simulink model "ACDCMG_woPV"  (R2020b)
settings: Solver=FixedStepAuto  StartTime=0.0  StopTime=0.2  FixedStep=Ts  MaxStep=1e-2  RelTol=1e-3
InitFcn:
  | Set_parameters_R2018
undefined symbols (not defined in the file): D1, D_invs, Delta, dis11, dis14, dis2, dis3, dis4, dis5, dis6, dis8, DiscIntNeverNeededParam, ee_sli_rtmsupport, fn, Fnom, gcbh, H_invs, Ion, Lithium, max_min, P_Load_3, P_nom_inv, Pnom_T1, Pnom_T2, Pnom_T3, Ql_Load_3, R_Load_9, R_Load_DC, Rl, Rls, S, sigbuilder_block, Ts, Ts_Control, Ts_Power, V1_LL_T3, VnInv, Vnom_DC, Vnom_Diesel, Vnom_prim, Vnom_sec, Vnom_ter_AC_DC, Xl, Xls
libraries: powerlib x238, powerlib_meascontrol x103, powerlib_extras x55, simulink x21, pid_lib x4, eeGeneralControl x2, re_lib x1, electricdrivelib x1, eeSinusoidalMeasurementV2 x1, eePowerMeasurement x1
(part 4 of 9)

== system ACDCMG_woPV/Resource1 ==
  note: http://calculationsolar.com/blog/?cat=2
  Constant1 : Constant  Value=max_min
  Irradiance (W/m^2) : Display
      settings: Format=bank  Decimation=1000
  Irradiance Temp Demand Max : Subsystem  Tag=STV Subsys  LoadFcn=sigbuilder_block('load');  StartFcn=sigbuilder_block('start');  StopFcn=sigbuilder_block('stop');  ClipboardFcn=sigbuilder_block('clipboard');  mask(Sigbuilder block){tuvar=[0:10]}
      mask help: Sigbuilder GUI
      mask init:
      | if ~strcmp(get_param(bdroot(gcbh),'SimulationStatus'),'stopped') tuvar = sigbuilder_block('maskInit'); end
      settings: CopyFcn=sigbuilder_block('copy');  DeleteFcn=sigbuilder_block('delete');  ModelCloseFcn=sigbuilder_block('modelClose');  PreSaveFcn=sigbuilder_block('preSave');  PauseFcn=sigbuilder_block('pause')  ContinueFcn=sigbuilder_block('continue')  NameChangeFcn=sigbuilder_block('namechange');  OpenFcn=sigbuilder_block('open',[0 30 1024.5 488.25 ]);  CloseFcn=sigbuilder_block('close');
      mask Display: plot(0, 0, 100, 100,[2, 2, 32, 32, 2], [68, 8, 8, 68, 68],[32, 2], [38, 38], [32, 19, 2],[53, 60, 44], [32, 17, 17, 2],[16, 16, 31, 31]);txt = getActiveGroup(gcbh);text(2, 100, txt,'verticalAlignment', 'top');
  Irradiance MIn Demand : Constant  Value=0
  Switch2 : Switch  Criteria=u2 > Threshold
  Temperature (deg. C) : Display
      settings: Format=bank  Decimation=1000
  Temp : Outport  VectorParamsAs1DForOutWhenUnconnected=off
  Ir : Outport  Port=2  VectorParamsAs1DForOutWhenUnconnected=off
  wires:
  Irradiance Temp Demand Max/1(Ir) -> Switch2/1, Irradiance (W/m^2)/1
  Irradiance Temp Demand Max/2(Temp) -> Temp/1, Temperature (deg. C)/1
  Irradiance MIn Demand/1 -> Switch2/3
  Constant1/1 -> Switch2/2
  Switch2/1 -> Ir/1  "Radiación (kW/m2)"

== system ACDCMG_woPV/Boost -buck Bi-directional converter 1 0.65 kW/+ve reference For Buck --> -ve reference For Boost <-- ==
  note: Buck PWM
  note: Duty Cycle
  note: Upper logic
  note: Lower logic
  note: Boost PWM
  note: Duty Cycle
  I_ref : Inport
  PID Orig Boost : Subsystem
  PID Orig Buck : Subsystem
  Relational Operator : RelationalOperator  Operator=>  OutDataTypeStr=boolean  RndMeth=Nearest
  Relational Operator1 : RelationalOperator  Operator=>  OutDataTypeStr=boolean  RndMeth=Nearest
  Saturation : Saturate  UpperLimit=0.9  LowerLimit=0
  Saturation1 : Saturate  UpperLimit=0.8  LowerLimit=0
  Sawtooth : simulink/Sources/Repeating Sequence  rep_seq_t=[0 1/5000]  rep_seq_y=[0 1]
  Sawtooth1 : simulink/Sources/Repeating Sequence  rep_seq_t=[0 1/5000]  rep_seq_y=[0 1]
  Sign : Gain  Gain=-1
  Sign1 : Gain  Gain=-1
  Sum : Sum  Inputs=|+-
  Sum2 : Sum  Inputs=-+|
  Switch : Switch  Criteria=u2 > Threshold
  Switch1 : Switch
  Vref1 : Constant  Value=0
  Vref2 : Constant  Value=0
  buck_I_Ctrl : Outport  VectorParamsAs1DForOutWhenUnconnected=off
  boost_I_Ctrl : Outport  Port=2  VectorParamsAs1DForOutWhenUnconnected=off
  wires:
  Sum/1 -> PID Orig Boost/1(error)  "error"
  Relational Operator/1 -> [boost1]
  Sign/1 -> Sum/1
  PID Orig Boost/1(Out1) -> Saturation/1
  PID Orig Buck/1(Out1) -> Saturation1/1
  Sawtooth/1 -> Relational Operator/2
  Sawtooth1/1 -> Relational Operator1/2
  Relational Operator1/1 -> [buck1]
  Sum2/1 -> PID Orig Buck/1(error)  "error"
  Saturation/1 -> Relational Operator/1
  Saturation1/1 -> Relational Operator1/1
  Vref1/1 -> Switch/3
  Vref2/1 -> Switch1/1
  [boost1] -> Switch1/3
  [buck1] -> Switch/1
  I_ref/1 -> Switch1/2, Switch/2, Sum2/2, Sign/1  "Current Reference"
  Sign1/1 -> Sum/2
  Switch1/1 -> boost_I_Ctrl/1
  Switch/1 -> buck_I_Ctrl/1
  [current] -> Sum2/1, Sign1/1

== system ACDCMG_woPV/Boost -buck Bi-directional converter 1 0.65 kW/OP_max // min ==
  boost_V_Ctrll : Inport
  buck_V_Ctrl : Inport  Port=2
  buck_I_Ctrl : Inport  Port=3
  boost_I_Ctrll : Inport  Port=4
  Control modes 0- Current 1- Coltage : Constant
  OP_max1 : Constant
  OP_min1 : Constant  Value=0
  Switch1 : Switch  Criteria=u2 > Threshold
  Switch2 : Switch  Criteria=u2 > Threshold
  Switch3 : Switch  Criteria=u2 > Threshold
  Op_Max / Min : Outport  VectorParamsAs1DForOutWhenUnconnected=off
  g_buck : Outport  Port=2  VectorParamsAs1DForOutWhenUnconnected=off
  g_boost : Outport  Port=3  VectorParamsAs1DForOutWhenUnconnected=off
  wires:
  OP_max1/1 -> Switch2/1
  OP_min1/1 -> Switch2/3
  Switch2/1 -> Op_Max / Min/1
  Control modes 0- Current 1- Coltage/1 -> Switch2/2, Switch1/2, Switch3/2
  boost_I_Ctrll/1 -> Switch1/3
  boost_V_Ctrll/1 -> Switch1/1
  buck_V_Ctrl/1 -> Switch3/1
  buck_I_Ctrl/1 -> Switch3/3
  Switch1/1 -> g_boost/1
  Switch3/1 -> g_buck/1

== system ACDCMG_woPV/Boost -buck Bi-directional converter 1 0.65 kW/Primary Control ==
  V_ref : Inport
  Constant : Constant
  Display3 : Display  Commented=on
  From1 : From  Commented=on  GotoTag=Vdc_bus  TagVisibility=global
  From4 : From  Commented=on  GotoTag=boost1
  From5 : From  Commented=on  GotoTag=buck1
  PID Orig Boost : Subsystem
  Relational Operator2 : RelationalOperator  Commented=on  Operator=>  OutDataTypeStr=boolean  RndMeth=Nearest
  Saturation : Saturate  UpperLimit=0.9  LowerLimit=0.1
  Scope1 : Scope
  Sum : Sum  Inputs=|+-
  Sum1 : Sum  Inputs=|-+
  Switch : Switch  Commented=on  Criteria=u2 > Threshold  Threshold=300
  Switch1 : Switch  Commented=on  Criteria=u2 > Threshold  Threshold=300
  Vref1 : Constant  Commented=on  Value=0
  Vref2 : Constant  Commented=on  Value=0
  Duty_Ctrl : Outport  VectorParamsAs1DForOutWhenUnconnected=off
  Comp_Duty_Ctrl : Outport  Port=2  VectorParamsAs1DForOutWhenUnconnected=off
  wires:
  Relational Operator2/1 -> Switch1/2, Switch/2
  V_ref/1 -> Sum/1, Relational Operator2/2
  From1/1 -> Relational Operator2/1
  Vref2/1 -> Switch1/1
  [Vdc_bus] -> Sum/2
  From5/1 -> Switch/1
  From4/1 -> Switch1/3
  Switch/1 -> Display3/1
  Vref1/1 -> Switch/3
  Sum/1 -> PID Orig Boost/1(error)  "error"
  PID Orig Boost/1(Out1) -> Saturation/1
  Constant/1 -> Sum1/2
  Saturation/1 -> Sum1/1, Duty_Ctrl/1, Scope1/1
  Sum1/1 -> Comp_Duty_Ctrl/1

== system ACDCMG_woPV/Boost -buck Bi-directional converter DC //CD 1 0.65 kW/+ve reference For Buck --> -ve reference For Boost <-- ==
  note: Notes :
      | 1- Saturation block : in practical applications during experiment, in the begining if the experiment, the error is usually high, therefore, duty cycle might reach value of 1, which means the IGBT switch will be shorted for a while which might cause damage to your circuit. it is preferable to put the saturation value to 0.7 during experiment, once you trust your circuit, you can increase up to 0.9.
      | 2- Sawtooth : We choose the frequancy of the sawtooth to be 5 kHz, because according to some papers if you go beyond this value, parastic elements will show up (i.e. its like an imaginary resistance and capcitance that causes switching losses and heat). But the more you increase the frequency, the smoother the signal you will get.
      | 3- Step size of your mode l: Make sure that the step size (sample time) in the "model configuration parameters" is smaller than 1/f of the sawtooth. For example, lets say that the sawtooth f = 2 Hz or cycle/sec, meaning the triangle (cycle) repeats every 1/2 sec. Step size or sample time means how many point matlab plot every cycle, lets say it is 1/4 (i.e. plot a point every 0.25 sec), that means that the triangle will be plotted with only two points. That reduce the accuracy, Moreover if the step size is greater than 1/f of the sawtooth, the sawtooth output will be zero.
  note: Buck PWM
  note: Duty Cycle
  note: Upper logic
  note: Lower logic
  note: Boost PWM
  note: Duty Cycle
  I_ref : Inport
  Display3 : Display
  Display4 : Display
  Integrator : Integrator  LimitOutput=on  UpperSaturationLimit=0.9  LowerSaturationLimit=0
  Integrator1 : Integrator  LimitOutput=on  UpperSaturationLimit=0.9  LowerSaturationLimit=0
  Ki : Gain  Gain=3
  Ki1 : Gain  Gain=110
  Kp : Gain  Gain=0.02
  Kp1 : Gain  Gain=0.2
  Relational Operator : RelationalOperator  Operator=>  OutDataTypeStr=boolean  RndMeth=Nearest
  Relational Operator1 : RelationalOperator  Operator=>  OutDataTypeStr=boolean  RndMeth=Nearest
  Saturation : Saturate  UpperLimit=0.9  LowerLimit=0
  Saturation1 : Saturate  UpperLimit=0.8  LowerLimit=0
  Sawtooth : simulink/Sources/Repeating Sequence  rep_seq_t=[0 1/5000]  rep_seq_y=[0 1]
  Sawtooth1 : simulink/Sources/Repeating Sequence  rep_seq_t=[0 1/5000]  rep_seq_y=[0 1]
  Sign : Gain  Gain=-1
  Sign1 : Gain  Gain=-1
  Sum : Sum  Inputs=|+-
  Sum1 : Sum  Inputs=|++
  Sum2 : Sum  Inputs=|+-
  Sum3 : Sum  Inputs=|++
  Switch : Switch  Criteria=u2 > Threshold
  Switch1 : Switch
  Vref1 : Constant  Value=0
  Vref2 : Constant  Value=0
  buck : Outport  VectorParamsAs1DForOutWhenUnconnected=off
  boost : Outport  Port=2  VectorParamsAs1DForOutWhenUnconnected=off
  tag scope: boost1=global, buck1=global
  wires:
  Integrator/1 -> Sum1/2
  Kp/1 -> Sum1/1
  Sum/1 -> Kp/1, Ki/1  "error"
  Relational Operator/1 -> [boost1]
  Sign/1 -> Sum/1
  Sum1/1 -> Saturation/1
  Ki/1 -> Integrator/1
  Sum3/1 -> Saturation1/1
  Integrator1/1 -> Sum3/2
  Sawtooth/1 -> Relational Operator/2
  Sawtooth1/1 -> Relational Operator1/2
  [current] -> Sum2/2, Sign1/1
  Kp1/1 -> Sum3/1
  Relational Operator1/1 -> [buck1]
  Sum2/1 -> Ki1/1, Kp1/1  "error"
  Saturation/1 -> Relational Operator/1
  Saturation1/1 -> Relational Operator1/1
  Ki1/1 -> Integrator1/1
  Vref1/1 -> Switch/3
  Vref2/1 -> Switch1/1
  [boost1] -> Switch1/3
  [buck1] -> Switch/1
  I_ref/1 -> Sum2/1, Sign/1, Switch1/2, Switch/2  "Current Reference"
  Sign1/1 -> Sum/2
  Switch1/1 -> Display4/1, boost/1
  Switch/1 -> Display3/1, buck/1

== system ACDCMG_woPV/Boost -buck Bi-directional converter DC //CD 1 0.65 kW/ref ==
  note: 1 -charge
      | 0-discharge
  Constant2 : Constant  Value=max_min
  Constant3 : Constant  Value=max_min
  Current reference (battery charge) OP_Max : Constant  Value=5
  Current reference (battery discharge) OP_Max1 : Constant  Value=-5
  Min Demand OP_min : Constant  Value=3
  Min Demand OP_min1 : Constant  Value=-3
  Switch : Switch  Criteria=u2 > Threshold
  Switch1 : Switch  Criteria=u2 > Threshold
  Switch3 : Switch  Criteria=u2 > Threshold
  Vref1 : Constant
  ref : Outport  VectorParamsAs1DForOutWhenUnconnected=off
  wires:
  Constant3/1 -> Switch3/2
  Switch3/1 -> Switch/3
  Switch1/1 -> Switch/1
  Vref1/1 -> Switch/2
  Min Demand OP_min/1 -> Switch1/3
  Current reference (battery charge) OP_Max/1 -> Switch1/1
  Min Demand OP_min1/1 -> Switch3/3
  Constant2/1 -> Switch1/2
  Current reference (battery discharge) OP_Max1/1 -> Switch3/1
  Switch/1 -> ref/1

== system ACDCMG_woPV/Boost -buck Bi-directional converter DC //DC 1 0.65 kW Switching Model/+ve reference For Buck --> -ve reference For Boost <-- ==
  note: Buck PWM
  note: Duty Cycle
  note: Upper logic
  note: Lower logic
  note: Boost PWM
  note: Duty Cycle
  I_ref : Inport
  PID Orig Boost : Subsystem
  PID Orig Buck : Subsystem
  Relational Operator : RelationalOperator  Operator=>  OutDataTypeStr=boolean  RndMeth=Nearest
  Relational Operator1 : RelationalOperator  Operator=>  OutDataTypeStr=boolean  RndMeth=Nearest
  Saturation : Saturate  UpperLimit=0.9  LowerLimit=0
  Saturation1 : Saturate  UpperLimit=0.8  LowerLimit=0
  Sawtooth : simulink/Sources/Repeating Sequence  rep_seq_t=[0 1/5000]  rep_seq_y=[0 1]
  Sawtooth1 : simulink/Sources/Repeating Sequence  rep_seq_t=[0 1/5000]  rep_seq_y=[0 1]
  Sign : Gain  Gain=-1
  Sign1 : Gain  Gain=-1
  Sum : Sum  Inputs=|+-
  Sum2 : Sum  Inputs=-+|
  Switch : Switch  Criteria=u2 > Threshold
  Switch1 : Switch
  Vref1 : Constant  Value=0
  Vref2 : Constant  Value=0
  buck_I_Ctrl : Outport  VectorParamsAs1DForOutWhenUnconnected=off
  boost_I_Ctrl : Outport  Port=2  VectorParamsAs1DForOutWhenUnconnected=off
  wires:
  Sum/1 -> PID Orig Boost/1(error)  "error"
  Relational Operator/1 -> [boost1]
  Sign/1 -> Sum/1
  PID Orig Boost/1(Out1) -> Saturation/1
  PID Orig Buck/1(Out1) -> Saturation1/1
  Sawtooth/1 -> Relational Operator/2
  Sawtooth1/1 -> Relational Operator1/2
  Relational Operator1/1 -> [buck1]
  Sum2/1 -> PID Orig Buck/1(error)  "error"
  Saturation/1 -> Relational Operator/1
  Saturation1/1 -> Relational Operator1/1
  Vref1/1 -> Switch/3
  Vref2/1 -> Switch1/1
  [boost1] -> Switch1/3
  [buck1] -> Switch/1
  I_ref/1 -> Switch1/2, Switch/2, Sum2/2, Sign/1  "Current Reference"
  Sign1/1 -> Sum/2
  Switch1/1 -> boost_I_Ctrl/1
  Switch/1 -> buck_I_Ctrl/1
  [current] -> Sum2/1, Sign1/1

== system ACDCMG_woPV/Boost -buck Bi-directional converter DC //DC 1 0.65 kW Switching Model/OP_max // min ==
  boost_V_Ctrll : Inport
  buck_V_Ctrl : Inport  Port=2
  buck_I_Ctrl : Inport  Port=3
  boost_I_Ctrll : Inport  Port=4
  Control modes 0- Current 1- Coltage : Constant
  OP_max1 : Constant
  OP_min1 : Constant  Value=0
  Switch1 : Switch  Criteria=u2 > Threshold
  Switch2 : Switch  Criteria=u2 > Threshold
  Switch3 : Switch  Criteria=u2 > Threshold
  Op_Max / Min : Outport  VectorParamsAs1DForOutWhenUnconnected=off
  g_buck : Outport  Port=2  VectorParamsAs1DForOutWhenUnconnected=off
  g_boost : Outport  Port=3  VectorParamsAs1DForOutWhenUnconnected=off
  wires:
  OP_max1/1 -> Switch2/1
  OP_min1/1 -> Switch2/3
  Switch2/1 -> Op_Max / Min/1
  Control modes 0- Current 1- Coltage/1 -> Switch2/2, Switch1/2, Switch3/2
  boost_I_Ctrll/1 -> Switch1/3
  boost_V_Ctrll/1 -> Switch1/1
  buck_V_Ctrl/1 -> Switch3/1
  buck_I_Ctrl/1 -> Switch3/3
  Switch1/1 -> g_boost/1
  Switch3/1 -> g_buck/1

== system ACDCMG_woPV/Boost -buck Bi-directional converter DC //DC 1 0.65 kW Switching Model/Primary Control ==
  V_ref : Inport
  Display3 : Display
  Display4 : Display
  PID Orig Boost : Subsystem
  PID Orig Buck : Subsystem
  Relational Operator : RelationalOperator  Operator=>  OutDataTypeStr=boolean  RndMeth=Nearest
  Relational Operator1 : RelationalOperator  Operator=>  OutDataTypeStr=boolean  RndMeth=Nearest
  Relational Operator2 : RelationalOperator  Operator=>  OutDataTypeStr=boolean  RndMeth=Nearest
  Repeating Sequence : simulink/Sources/Repeating Sequence  rep_seq_t=[0 1/5000]  rep_seq_y=[0 1]
  Repeating Sequence1 : simulink/Sources/Repeating Sequence  rep_seq_t=[0 1/5000]  rep_seq_y=[0 1]
  Saturation : Saturate  UpperLimit=0.9  LowerLimit=0
  Saturation1 : Saturate  UpperLimit=0.9  LowerLimit=0
  Sum : Sum  Inputs=|+-
  Sum2 : Sum  Inputs=|+-
  Switch : Switch  Criteria=u2 > Threshold  Threshold=300
  Switch1 : Switch  Criteria=u2 > Threshold  Threshold=300
  Vref1 : Constant  Value=0
  Vref2 : Constant  Value=0
  buck_V_Ctrl : Outport  VectorParamsAs1DForOutWhenUnconnected=off
  boost_V_Ctrl : Outport  Port=2  VectorParamsAs1DForOutWhenUnconnected=off
  wires:
  Relational Operator2/1 -> Switch1/2, Switch/2
  Saturation1/1 -> Relational Operator1/1
  V_ref/1 -> Sum/1, Relational Operator2/2, Sum2/1
  [Vdc_bus] -> Relational Operator2/1
  Vref2/1 -> Switch1/1
  Repeating Sequence/1 -> Relational Operator/2
  Repeating Sequence1/1 -> Relational Operator1/2
  Relational Operator1/1 -> [buck1]
  [Vdc_bus] -> Sum2/2, Sum/2
  [buck1] -> Switch/1
  Switch1/1 -> Display4/1, boost_V_Ctrl/1
  Saturation/1 -> Relational Operator/1
  [boost1] -> Switch1/3
  Sum2/1 -> PID Orig Buck/1(error)  "error"
  Relational Operator/1 -> [boost1]
  Switch/1 -> Display3/1, buck_V_Ctrl/1
  Vref1/1 -> Switch/3
  Sum/1 -> PID Orig Boost/1(error)  "error"
  PID Orig Buck/1(Out1) -> Saturation1/1
  PID Orig Boost/1(Out1) -> Saturation/1

== system ACDCMG_woPV/Boost converter DC //CD 2 5 kHz - 300V /MPPT Controller using  "Incremental Conductance + Integral Regulator "  technique  ==
  note: +
  note: control mppt
  V_PV : Inport
  I_PV : Inport  Port=2
  Add : Sum  Inputs=+-
  Deblock MPPT : Step  Time=0.2  SampleTime=0
  Duty Cycle : Constant  Value=Dinit
  MPPT : Subsystem
  PWM Generator (DC-DC) : powerlib_meascontrol/Pulse & Signal Generators/PWM Generator (DC-DC)  Fsw=fc  Ts=Ts_Power
  Saturation : Saturate  UpperLimit=1  LowerLimit=0
  Pulses : Outport  VectorParamsAs1DForOutWhenUnconnected=off
  tag scope: D=global
  wires:
  V_PV/1 -> MPPT/1(V_PV)
  I_PV/1 -> MPPT/2(I_PV)
  PWM Generator (DC-DC)/1 -> Pulses/1
  Deblock MPPT/1 -> MPPT/3(on/off)
  Add/1 -> Saturation/1  "D"
  MPPT/1(Delta_D) -> Add/2  "Vdc_ref"
  Duty Cycle/1 -> Add/1
  Saturation/1 -> [D], PWM Generator (DC-DC)/1

== system ACDCMG_woPV/Boost converter DC //CD 2 5 kHz - 300V 1/MPPT Controller using  "Incremental Conductance + Integral Regulator "  technique  ==
  note: +
  note: control mppt
  V_PV : Inport
  I_PV : Inport  Port=2
  Add : Sum  Inputs=+-
  Deblock MPPT : Step  Time=0.2  SampleTime=0
  Duty Cycle : Constant  Value=Dinit
  MPPT : Subsystem
  PWM Generator (DC-DC) : powerlib_meascontrol/Pulse & Signal Generators/PWM Generator (DC-DC)  Fsw=fc  Ts=Ts_Power
  Saturation : Saturate  UpperLimit=1  LowerLimit=0
  Pulses : Outport  VectorParamsAs1DForOutWhenUnconnected=off
  tag scope: D=global
  wires:
  V_PV/1 -> MPPT/1(V_PV)
  I_PV/1 -> MPPT/2(I_PV)
  PWM Generator (DC-DC)/1 -> Pulses/1
  Deblock MPPT/1 -> MPPT/3(on/off)
  Add/1 -> Saturation/1  "D"
  MPPT/1(Delta_D) -> Add/2  "Vdc_ref"
  Duty Cycle/1 -> Add/1
  Saturation/1 -> [D], PWM Generator (DC-DC)/1

== system ACDCMG_woPV/Boost converter DC //DC 2 5 kHz - 300V /  ==
  V_PV : Inport
  I_PV : Inport  Port=2
  Duty Cycle : Constant  Value=0.34
  PWM Generator (DC-DC) : powerlib_meascontrol/Pulse & Signal Generators/PWM Generator (DC-DC)  Fsw=fc  Ts=Ts_Power
  Terminator1 : Terminator
  Terminator2 : Terminator
  Pulses : Outport  VectorParamsAs1DForOutWhenUnconnected=off
  tag scope: D=global
  wires:
  V_PV/1 -> Terminator1/1
  I_PV/1 -> Terminator2/1
  PWM Generator (DC-DC)/1 -> Pulses/1
  Duty Cycle/1 -> [D], PWM Generator (DC-DC)/1

== system ACDCMG_woPV/Bus_1/Power Factor Block1 ==
  Vabc : Inport
  Iabc : Inport  Port=2
  Complex to Magnitude-Angle : ComplexToMagnitudeAngle  Commented=on
  Conv pu1 : Gain  Gain=sqrt (3) /Vnom_sec  SaturateOnIntegerOverflow=on  OutDataTypeStr=Inherit: Same as input  ParamDataTypeStr=Inherit: Same as input
  Current1 : Goto  Commented=on  GotoTag=P_abc_Bus1  TagVisibility=global
  Current2 : Goto  Commented=on  GotoTag=Q_abc_Bus1  TagVisibility=global
  Gain1 : Gain  Commented=on  Gain=-1/1000
  Mux : Mux  Inputs=2
  Power : powerlib_meascontrol/Measurements/Power  Commented=on  Freq=Freq  Vinit=Vinit  Iinit=Iinit  Ts=Ts
  Real-Imag to Complex : RealImagToComplex  Commented=on
  Terminator : Terminator  Commented=on
  cos(theta) : Trigonometry  Commented=on  Operator=cos
  to Kw : Gain  Commented=on  Gain=-1/1000
  "Vabc y Vabc " : Outport  VectorParamsAs1DForOutWhenUnconnected=off
  "Iabc y Iabc " : Outport  Port=2  VectorParamsAs1DForOutWhenUnconnected=off
  tag scope: Vabc_LL_pu_Bus1=global
  wires:
  Power/1 -> Gain1/1, Real-Imag to Complex/1
  Power/2 -> Real-Imag to Complex/2, to Kw/1
  Complex to Magnitude-Angle/2 -> cos(theta)/1
  Real-Imag to Complex/1 -> Complex to Magnitude-Angle/1
  Complex to Magnitude-Angle/1 -> Terminator/1
  Iabc/1 -> "Iabc y Iabc "/1, Power/2
  Mux/1 -> "Vabc y Vabc "/1
  Vabc/1 -> Power/1, Conv pu1/1, Mux/1, Mux/2
  Conv pu1/1 -> [Vabc_LL_pu_Bus1]
  to Kw/1 -> Current2/1
  Gain1/1 -> Current1/1

== system ACDCMG_woPV/Bus_2/Power Factor Block1 ==
  Vabc : Inport
  Iabc : Inport  Port=2
  Complex to Magnitude-Angle : ComplexToMagnitudeAngle  Commented=on
  Conv pu1 : Gain  Gain=sqrt (3) /Vnom_sec  SaturateOnIntegerOverflow=on  OutDataTypeStr=Inherit: Same as input  ParamDataTypeStr=Inherit: Same as input
  Current3 : Goto  Commented=on  GotoTag=P_abc_Bus2  TagVisibility=global
  Current4 : Goto  Commented=on  GotoTag=Q_abc_Bus2  TagVisibility=global
  Mux : Mux  Inputs=2
  Power : powerlib_meascontrol/Measurements/Power  Commented=on  Freq=Freq  Vinit=Vinit  Iinit=Iinit  Ts=Ts
  Real-Imag to Complex : RealImagToComplex  Commented=on
  Terminator : Terminator  Commented=on
  cos(theta) : Trigonometry  Commented=on  Operator=cos
  to Kw : Gain  Commented=on  Gain=-1/1000
  to Kw1 : Gain  Commented=on  Gain=-1/1000
  "Vabc y Vabc " : Outport  VectorParamsAs1DForOutWhenUnconnected=off
  Iabc y Iabc : Outport  Port=2  VectorParamsAs1DForOutWhenUnconnected=off
  tag scope: Vabc_LL_pu_Bus2=global
  wires:
  Complex to Magnitude-Angle/2 -> cos(theta)/1
  Real-Imag to Complex/1 -> Complex to Magnitude-Angle/1
  cos(theta)/1 -> ?
  Complex to Magnitude-Angle/1 -> Terminator/1
  Iabc/1 -> Iabc y Iabc/1, Power/2
  Mux/1 -> "Vabc y Vabc "/1
  Vabc/1 -> Power/1, Conv pu1/1, Mux/1, Mux/2
  Conv pu1/1 -> [Vabc_LL_pu_Bus2]
  Power/1 -> to Kw1/1, Real-Imag to Complex/1
  Power/2 -> to Kw/1, Real-Imag to Complex/2
  to Kw/1 -> Current4/1
  to Kw1/1 -> Current3/1

== system ACDCMG_woPV/Bus_3 /Power Factor Block1 ==
  Vabc : Inport
  Iabc : Inport  Port=2
  Complex to Magnitude-Angle : ComplexToMagnitudeAngle  Commented=on
  Conv pu2 : Gain  Gain=sqrt (3) /Vnom_prim  SaturateOnIntegerOverflow=on  OutDataTypeStr=Inherit: Same as input  ParamDataTypeStr=Inherit: Same as input
  Current3 : Goto  Commented=on  GotoTag=P_abc_Bus3  TagVisibility=global
  Current4 : Goto  Commented=on  GotoTag=Q_abc_Bus3  TagVisibility=global
  Gain : Gain  Commented=on  Gain=-1/1000
  Gain1 : Gain  Commented=on  Gain=-1/1000
  Mux : Mux  Inputs=2
  Power : powerlib_meascontrol/Measurements/Power  Commented=on  Freq=Freq  Vinit=Vinit  Iinit=Iinit  Ts=Ts
  Real-Imag to Complex : RealImagToComplex  Commented=on
  Terminator : Terminator  Commented=on
  cos(theta) : Trigonometry  Commented=on  Operator=cos
  "Vabc y Vabc " : Outport  VectorParamsAs1DForOutWhenUnconnected=off
  "Iabc y Iabc " : Outport  Port=2  VectorParamsAs1DForOutWhenUnconnected=off
  tag scope: Vabc_LL_pu_Bus3=global
  wires:
  Complex to Magnitude-Angle/2 -> cos(theta)/1
  Real-Imag to Complex/1 -> Complex to Magnitude-Angle/1
  cos(theta)/1 -> ?
  Complex to Magnitude-Angle/1 -> Terminator/1
  Iabc/1 -> "Iabc y Iabc "/1, Power/2
  Mux/1 -> "Vabc y Vabc "/1
  Vabc/1 -> Power/1, Conv pu2/1, Mux/1, Mux/2
  Conv pu2/1 -> [Vabc_LL_pu_Bus3]
  Power/1 -> Gain/1, Real-Imag to Complex/1
  Power/2 -> Real-Imag to Complex/2, Gain1/1
  Gain1/1 -> Current4/1
  Gain/1 -> Current3/1

== system ACDCMG_woPV/Bus_4/Power Factor Block1 ==
  Vabc : Inport
  Iabc : Inport  Port=2
  Complex to Magnitude-Angle : ComplexToMagnitudeAngle  Commented=on
  Conv pu1 : Gain  Gain=sqrt (3) /Vnom_sec  SaturateOnIntegerOverflow=on  OutDataTypeStr=Inherit: Same as input  ParamDataTypeStr=Inherit: Same as input
  Current3 : Goto  Commented=on  GotoTag=P_abc_Bus4  TagVisibility=global
  Current4 : Goto  Commented=on  GotoTag=Q_abc_Bus4  TagVisibility=global
  Mux : Mux  Inputs=2
  Power : powerlib_meascontrol/Measurements/Power  Commented=on  Freq=Freq  Vinit=Vinit  Iinit=Iinit  Ts=Ts
  Real-Imag to Complex : RealImagToComplex  Commented=on
  Terminator : Terminator  Commented=on
  cos(theta) : Trigonometry  Commented=on  Operator=cos
  to Kw : Gain  Commented=on  Gain=1/1000
  to Kw1 : Gain  Commented=on  Gain=1/1000
  Vabc y Vabc : Outport  VectorParamsAs1DForOutWhenUnconnected=off
  "Iabc y Iabc " : Outport  Port=2  VectorParamsAs1DForOutWhenUnconnected=off
  tag scope: Vabc_LL_pu_Bus4=global
  wires:
  Complex to Magnitude-Angle/2 -> cos(theta)/1
  Real-Imag to Complex/1 -> Complex to Magnitude-Angle/1
  cos(theta)/1 -> ?
  Complex to Magnitude-Angle/1 -> Terminator/1
  Iabc/1 -> "Iabc y Iabc "/1, Power/2
  Mux/1 -> Vabc y Vabc/1
  Conv pu1/1 -> [Vabc_LL_pu_Bus4]
  Vabc/1 -> Power/1, Conv pu1/1, Mux/1, Mux/2
  Power/2 -> Real-Imag to Complex/2, to Kw/1
  Power/1 -> to Kw1/1, Real-Imag to Complex/1
  to Kw/1 -> Current4/1
  to Kw1/1 -> Current3/1

== system ACDCMG_woPV/Bus_5/Power Factor Block1 ==
  Vabc : Inport
  Iabc : Inport  Port=2
  Complex to Magnitude-Angle : ComplexToMagnitudeAngle  Commented=on
  Conv pu1 : Gain  Gain=sqrt (3) /Vnom_sec  SaturateOnIntegerOverflow=on  OutDataTypeStr=Inherit: Same as input  ParamDataTypeStr=Inherit: Same as input
  Current3 : Goto  Commented=on  GotoTag=P_abc_Bus5  TagVisibility=global
  Current4 : Goto  Commented=on  GotoTag=Q_abc_Bus5  TagVisibility=global
  Mux : Mux  Inputs=2
  Power : powerlib_meascontrol/Measurements/Power  Commented=on  Freq=Freq  Vinit=Vinit  Iinit=Iinit  Ts=Ts
  Real-Imag to Complex : RealImagToComplex  Commented=on
  Terminator : Terminator  Commented=on
  cos(theta) : Trigonometry  Commented=on  Operator=cos
  to Kw : Gain  Commented=on  Gain=1/1000
  to Kw1 : Gain  Commented=on  Gain=1/1000
  Vabc y Vabc : Outport  VectorParamsAs1DForOutWhenUnconnected=off
  "Iabc y Iabc " : Outport  Port=2  VectorParamsAs1DForOutWhenUnconnected=off
  tag scope: Vabc_LL_pu_Bus5=global
  wires:
  Complex to Magnitude-Angle/2 -> cos(theta)/1
  Real-Imag to Complex/1 -> Complex to Magnitude-Angle/1
  cos(theta)/1 -> ?
  Complex to Magnitude-Angle/1 -> Terminator/1
  Iabc/1 -> "Iabc y Iabc "/1, Power/2
  Mux/1 -> Vabc y Vabc/1
  Conv pu1/1 -> [Vabc_LL_pu_Bus5]
  Vabc/1 -> Power/1, Conv pu1/1, Mux/1, Mux/2
  Power/2 -> Real-Imag to Complex/2, to Kw/1
  Power/1 -> to Kw1/1, Real-Imag to Complex/1
  to Kw/1 -> Current4/1
  to Kw1/1 -> Current3/1

== system ACDCMG_woPV/Bus_6/Power Factor Block1 ==
  Vabc : Inport
  Iabc : Inport  Port=2
  Complex to Magnitude-Angle : ComplexToMagnitudeAngle  Commented=on
  Conv pu2 : Gain  Gain=sqrt (3) /Vnom_prim  SaturateOnIntegerOverflow=on  OutDataTypeStr=Inherit: Same as input  ParamDataTypeStr=Inherit: Same as input
  Current3 : Goto  Commented=on  GotoTag=P_abc_Bus6  TagVisibility=global
  Current4 : Goto  Commented=on  GotoTag=Q_abc_Bus6  TagVisibility=global
  Mux : Mux  Inputs=2
  Power : powerlib_meascontrol/Measurements/Power  Commented=on  Freq=Freq  Vinit=Vinit  Iinit=Iinit  Ts=Ts
  Real-Imag to Complex : RealImagToComplex  Commented=on
  Terminator : Terminator  Commented=on
  cos(theta) : Trigonometry  Commented=on  Operator=cos
  to Kw : Gain  Commented=on  Gain=1/1000
  to Kw1 : Gain  Commented=on  Gain=1/1000
  "Vabc y Vabc " : Outport  VectorParamsAs1DForOutWhenUnconnected=off
  "Iabc y Iabc " : Outport  Port=2  VectorParamsAs1DForOutWhenUnconnected=off
  tag scope: Vabc_LL_pu_Bus6=global
  wires:
  Complex to Magnitude-Angle/2 -> cos(theta)/1
  Real-Imag to Complex/1 -> Complex to Magnitude-Angle/1
  cos(theta)/1 -> ?
  Complex to Magnitude-Angle/1 -> Terminator/1
  Iabc/1 -> "Iabc y Iabc "/1, Power/2
  Mux/1 -> "Vabc y Vabc "/1
  Vabc/1 -> Power/1, Conv pu2/1, Mux/1, Mux/2
  Conv pu2/1 -> [Vabc_LL_pu_Bus6]
  Power/2 -> Real-Imag to Complex/2, to Kw/1
  Power/1 -> to Kw1/1, Real-Imag to Complex/1
  to Kw/1 -> Current4/1
  to Kw1/1 -> Current3/1

== system ACDCMG_woPV/Bus_7/Power Factor Block1 ==
  Vabc : Inport
  Iabc : Inport  Port=2
  Complex to Magnitude-Angle : ComplexToMagnitudeAngle  Commented=on
  Conv pu2 : Gain  Gain=sqrt (3) /Vnom_prim  SaturateOnIntegerOverflow=on  OutDataTypeStr=Inherit: Same as input  ParamDataTypeStr=Inherit: Same as input
  Current3 : Goto  Commented=on  GotoTag=P_abc_Bus7  TagVisibility=global
  Current4 : Goto  Commented=on  GotoTag=Q_abc_Bus7  TagVisibility=global
  Mux : Mux  Inputs=2
  Power : powerlib_meascontrol/Measurements/Power  Commented=on  Freq=Freq  Vinit=Vinit  Iinit=Iinit  Ts=Ts
  Real-Imag to Complex : RealImagToComplex  Commented=on
  Terminator : Terminator  Commented=on
  cos(theta) : Trigonometry  Commented=on  Operator=cos
  to Kw : Gain  Commented=on  Gain=1/1000
  to Kw1 : Gain  Commented=on  Gain=1/1000
  "Vabc y Vabc " : Outport  VectorParamsAs1DForOutWhenUnconnected=off
  "Iabc y Iabc " : Outport  Port=2  VectorParamsAs1DForOutWhenUnconnected=off
  tag scope: Vabc_LL_pu_Bus7=global
  wires:
  Complex to Magnitude-Angle/2 -> cos(theta)/1
  Real-Imag to Complex/1 -> Complex to Magnitude-Angle/1
  cos(theta)/1 -> ?
  Complex to Magnitude-Angle/1 -> Terminator/1
  Iabc/1 -> "Iabc y Iabc "/1, Power/2
  Mux/1 -> "Vabc y Vabc "/1
  Conv pu2/1 -> [Vabc_LL_pu_Bus7]
  Vabc/1 -> Power/1, Conv pu2/1, Mux/1, Mux/2
  Power/2 -> Real-Imag to Complex/2, to Kw/1
  Power/1 -> to Kw1/1, Real-Imag to Complex/1
  to Kw/1 -> Current4/1
  to Kw1/1 -> Current3/1

== system ACDCMG_woPV/Bus_8      /Power Factor Block1 ==
  Vabc : Inport
  Iabc : Inport  Port=2
  Complex to Magnitude-Angle : ComplexToMagnitudeAngle  Commented=on
  Conv pu2 : Gain  Gain=sqrt (3) /Vnom_Diesel  SaturateOnIntegerOverflow=on  OutDataTypeStr=Inherit: Same as input  ParamDataTypeStr=Inherit: Same as input
  Current3 : Goto  Commented=on  GotoTag=P_abc_Bus8  TagVisibility=global
  Current4 : Goto  Commented=on  GotoTag=Q_abc_Bus8  TagVisibility=global
  Gain : Gain  Commented=on  Gain=-1/1000
  Gain1 : Gain  Commented=on  Gain=-1/1000
  Mux : Mux  Inputs=2
  Power : powerlib_meascontrol/Measurements/Power  Commented=on  Freq=Freq  Vinit=Vinit  Iinit=Iinit  Ts=Ts
  Real-Imag to Complex : RealImagToComplex  Commented=on
  Terminator : Terminator  Commented=on
  cos(theta) : Trigonometry  Commented=on  Operator=cos
  "Vabc y Vabc " : Outport  VectorParamsAs1DForOutWhenUnconnected=off
  "Iabc y Iabc " : Outport  Port=2  VectorParamsAs1DForOutWhenUnconnected=off
  tag scope: Vabc_LL_pu_Bus8=global
  wires:
  Complex to Magnitude-Angle/2 -> cos(theta)/1
  Real-Imag to Complex/1 -> Complex to Magnitude-Angle/1
  cos(theta)/1 -> ?
  Complex to Magnitude-Angle/1 -> Terminator/1
  Iabc/1 -> "Iabc y Iabc "/1, Power/2
  Mux/1 -> "Vabc y Vabc "/1
  Conv pu2/1 -> [Vabc_LL_pu_Bus8]
  Vabc/1 -> Power/1, Conv pu2/1, Mux/1, Mux/2
  Power/2 -> Real-Imag to Complex/2, Gain/1
  Power/1 -> Gain1/1, Real-Imag to Complex/1
  Gain/1 -> Current4/1
  Gain1/1 -> Current3/1

== system ACDCMG_woPV/Bus_9/Power Factor Block1 ==
  Vabc : Inport
  Iabc : Inport  Port=2
  Complex to Magnitude-Angle : ComplexToMagnitudeAngle  Commented=on
  Conv pu1 : Gain  Gain=sqrt (3) /Vnom_prim  SaturateOnIntegerOverflow=on  OutDataTypeStr=Inherit: Same as input  ParamDataTypeStr=Inherit: Same as input
  Current1 : Goto  Commented=on  GotoTag=P_abc_Bus9  TagVisibility=global
  Current2 : Goto  Commented=on  GotoTag=Q_abc_Bus9  TagVisibility=global
  Gain1 : Gain  Commented=on  Gain=-1/1000
  Mux : Mux  Inputs=2
  Power : powerlib_meascontrol/Measurements/Power  Commented=on  Freq=Freq  Vinit=Vinit  Iinit=Iinit  Ts=Ts
  Real-Imag to Complex : RealImagToComplex  Commented=on
  Terminator : Terminator  Commented=on
  cos(theta) : Trigonometry  Commented=on  Operator=cos
  to Kw : Gain  Commented=on  Gain=-1/1000
  "Vabc y Vabc " : Outport  VectorParamsAs1DForOutWhenUnconnected=off
  "Iabc y Iabc " : Outport  Port=2  VectorParamsAs1DForOutWhenUnconnected=off
  tag scope: Vabc_LL_pu_Bus9=global
  wires:
  Power/1 -> Gain1/1, Real-Imag to Complex/1
  Power/2 -> Real-Imag to Complex/2, to Kw/1
  Complex to Magnitude-Angle/2 -> cos(theta)/1
  Real-Imag to Complex/1 -> Complex to Magnitude-Angle/1
  cos(theta)/1 -> ?
  Complex to Magnitude-Angle/1 -> Terminator/1
  Iabc/1 -> "Iabc y Iabc "/1, Power/2
  Mux/1 -> "Vabc y Vabc "/1
  Vabc/1 -> Power/1, Conv pu1/1, Mux/1, Mux/2
  Conv pu1/1 -> [Vabc_LL_pu_Bus9]
  to Kw/1 -> Current2/1
  Gain1/1 -> Current1/1

== system ACDCMG_woPV/Bus_AC//DC3/Battery system ==
  note: DC Bus
  note: Bettery
  "0 = Enable (Do it after transient, so that it does not calculate ripples during transient) 1 = Reset after every change in current reference" : Constant  Value=0
  Current Inst : Scope
  Current going to/ from the battery : Scope
  Display6 : Display
  Mean : powerlib_meascontrol/Measurements/Mean  Freq=10  Vinit=0  Ts=0
  Power : Product
  Power Bess : Scope
  Ripple Calculations : Subsystem
  Ripple in Boost : Display
  Ripple in Buck : Display
  Vbat : Scope
  Vdc : Scope
  to Kw : Gain  Gain=1/1000
  wires:
  to Kw/1 -> Display6/1, Power Bess/1
  Mean/1 -> Power/2
  Power/1 -> to Kw/1
  Ripple Calculations/1(Ripple in Buck) -> Ripple in Buck/1
  "0 = Enable (Do it after transient, so that it does not calculate ripples during transient) 1 = Reset after every change in current reference"/1 -> Ripple Calculations/2(Reset)
  Ripple Calculations/2(Ripple in Boost) -> Ripple in Boost/1
  [Idc_bus] -> Mean/1, Ripple Calculations/1(Signal), Current Inst/1
  [current] -> Current going to/ from the battery/1
  [Vdc_bus] -> Vdc/1, Power/1
  [Vdc_battery] -> Vbat/1

== system ACDCMG_woPV/Bus_AC//DC3/PV system ==
  note: Bus DC
  note: PV
  Bus Selector : BusSelector  OutputSignals=V_PV,I_PV,I_diode,Irradiance (W/m2),Temperature (deg C)
  Current going to/ DC bus : Scope
  "P (kW) " : Display
      settings: Format=bank  Decimation=2000
  PV : Scope  NumInputPorts=3
  PV1 : Scope  NumInputPorts=5
  Pmean : Subsystem
  Vdc Boost : Display
      settings: Format=bank  Decimation=2000
  Vdc DC bus : Scope
  tag scope: I_PV=global, Idiode_PV=global, Ir=global, Temp=global, V_PV=global
  wires:
  [V_PV] -> PV/1  "V_PV"
  [I_PV] -> PV/2  "I_PV"
  [Idiode_PV] -> PV/3  "Idiode_PV"
  [m_PV] -> Bus Selector/1
  Bus Selector/1 -> [V_PV]  "<V_PV>"
  Bus Selector/2 -> [I_PV]  "<I_PV>"
  Bus Selector/4 -> [Ir]  "<Irradiance (W/m2)>"
  Bus Selector/3 -> [Idiode_PV]  "<I_diode>"
  Bus Selector/5 -> [Temp]  "<Temperature (deg C)>"
  [Temp] -> PV1/2  "Temp (deg. C)"
  [D] -> PV1/5  "Duty Cycle"
  Pmean/2(V) -> Vdc Boost/1, PV1/4  "Vmean (V)"
  [Ir] -> PV1/1  "Ir (W/m^2)"
  Pmean/1(P) -> "P (kW) "/1, PV1/3  "Pmean  (kW)"
  [I_DC_bus_PV] -> Current going to/ DC bus/1
  [V_DC_bus_PV] -> Vdc DC bus/1

== system ACDCMG_woPV/Bus_AC//DC4/Power Factor Block1 ==
  Vabc : Inport
  Iabc : Inport  Port=2
  Complex to Magnitude-Angle : ComplexToMagnitudeAngle  Commented=on
  Power : powerlib_meascontrol/Measurements/Power  Commented=on  Freq=Freq  Vinit=Vinit  Iinit=Iinit  Ts=Ts
  Real-Imag to Complex : RealImagToComplex  Commented=on
  Terminator : Terminator  Commented=on
  cos(theta) : Trigonometry  Commented=on  Operator=cos
  "Vabc y Vabc " : Outport  VectorParamsAs1DForOutWhenUnconnected=off
  "Iabc y Iabc " : Outport  Port=2  VectorParamsAs1DForOutWhenUnconnected=off
  wires:
  Power/1 -> Real-Imag to Complex/1
  Power/2 -> Real-Imag to Complex/2
  Complex to Magnitude-Angle/2 -> cos(theta)/1
  Real-Imag to Complex/1 -> Complex to Magnitude-Angle/1
  cos(theta)/1 -> ?
  Complex to Magnitude-Angle/1 -> Terminator/1
  Iabc/1 -> "Iabc y Iabc "/1, Power/2
  Vabc/1 -> "Vabc y Vabc "/1, Power/1

== system ACDCMG_woPV/Bus_AC//DC5/Power Factor Block1 ==
  Vabc : Inport
  Iabc : Inport  Port=2
  Complex to Magnitude-Angle : ComplexToMagnitudeAngle  Commented=on
  Power : powerlib_meascontrol/Measurements/Power  Commented=on  Freq=Freq  Vinit=Vinit  Iinit=Iinit  Ts=Ts
  Real-Imag to Complex : RealImagToComplex  Commented=on
  Terminator : Terminator  Commented=on
  cos(theta) : Trigonometry  Commented=on  Operator=cos
  "Vabc y Vabc " : Outport  VectorParamsAs1DForOutWhenUnconnected=off
  "Iabc y Iabc " : Outport  Port=2  VectorParamsAs1DForOutWhenUnconnected=off
  wires:
  Power/1 -> Real-Imag to Complex/1
  Power/2 -> Real-Imag to Complex/2
  Complex to Magnitude-Angle/2 -> cos(theta)/1
  Real-Imag to Complex/1 -> Complex to Magnitude-Angle/1
  cos(theta)/1 -> ?
  Complex to Magnitude-Angle/1 -> Terminator/1
  Iabc/1 -> "Iabc y Iabc "/1, Power/2
  Vabc/1 -> Power/1, "Vabc y Vabc "/1

== system ACDCMG_woPV/DATA  ADQUISITION/Power_Losses_abc ==
  From10 : From  Commented=on  GotoTag=Power_Losse_abc_L10  TagVisibility=global
  From11 : From  Commented=on  GotoTag=Power_Losse_abc_L10
  From12 : From  Commented=on  GotoTag=Power_Losse_abc_L12
  From13 : From  Commented=on  GotoTag=Power_Losse_abc_L14
  From6 : From  Commented=on  GotoTag=Power_Losse_abc_L3  TagVisibility=global
  Mux : Mux  Inputs=9
  f2 : ToWorkspace  VariableName=Power_Losse_abc  SaveFormat=Timeseries  SampleTime=-1
  wires:
  [Power_Losse_abc_L1] -> Mux/1
  Mux/1 -> f2/1
  [Power_Losse_abc_L2] -> Mux/2
  [Power_Losse_abc_L5] -> Mux/5
  [Power_Losse_abc_L6] -> Mux/6
  [Power_Losse_abc_L7] -> Mux/7
  [Power_Losse_abc_L3] -> Mux/3
  [Power_Losse_abc_L4] -> Mux/4
  [Power_Losse_abc_L8] -> Mux/8
  [Power_Losse_abc_L9] -> Mux/9

== system ACDCMG_woPV/DATA  ADQUISITION/VoltageLL_pu_abc ==
  From28 : From  Commented=on  GotoTag=Vabc_LL_pu_Bus10
  From31 : From  Commented=on  GotoTag=Vabc_LL_pu_Bus10
  From34 : From  Commented=on  GotoTag=Vabc_LL_pu_Bus12
  From40 : From  Commented=on  GotoTag=Vabc_LL_pu_Bus14
  Mux : Mux  Inputs=10
  f2 : ToWorkspace  VariableName=VoltageLL_pu_abc  SaveFormat=Timeseries  SampleTime=-1
  wires:
  [Vabc_LL_pu_Bus4] -> Mux/4
  [Vabc_LL_pu_Bus5] -> Mux/5
  Mux/1 -> f2/1
  [Vabc_LL_pu_Bus8] -> Mux/8
  [Vabc_LL_pu_Bus1] -> Mux/1
  [Vabc_LL_pu_Bus2] -> Mux/2
  [Vabc_LL_pu_Bus6] -> Mux/6
  [Vabc_LL_pu_Bus7] -> Mux/7
  [V_pu_BusDC] -> Mux/10
  [Vabc_LL_pu_Bus3] -> Mux/3
  [Vabc_LL_pu_Bus9] -> Mux/9

== system ACDCMG_woPV/Grid Bi-directional Converter 1.1 300 (DC) // 150 V (AC) P_nom 3kW/Control of Inverter ==
  note: VL-L rms_1
  note: Primary control
  note: Control of Inverter
  Means : Inport
  Bus Selector : BusSelector  OutputSignals=signal1,signal2,signal3,signal4
  Discrete PWM Generator1 : Subsystem  AncestorBlock=|  DialogController=POWERSYS.PowerSysDialog  mask(Discrete PWM Generator){GeneratorMode=3-arm  bridge (6 pulses), Fc=4000, Ts=Ts_Power, Internal=off, mIndex=0.99, Freq=60, Phase=0}
      | powerlib_extras/Discrete 
      | Control Blocks/Discrete
      | PWM Generator
      mask prompts: GeneratorMode "Generator Mode"; Fc "Carrier frequency (Hz):"; Ts "Sample time:"; Internal "Internal generation of modulating signal(s)"; mIndex "Modulation index  (0<m<1) :"; Freq "Frequency of output voltage (Hz)"; Phase "Phase of output voltage (degrees)"
      mask help:
      | This discrete block generates pulses for carrier-based PWM (Pulse Width Modulation), self-commutated IGBTs,GTOs or FETs bridges.
      |
      | Depending on the number of bridge arms selected in the "Generator Mode" parameter, the block can be used either for single-phase or three-phase PWM control.
      mask init:
      | powericon('psbcallbacks',gcb,'Discrete PWM Generator');
      | if Freq==0
      |     Phase=90;
      | end
      | switch GeneratorMode
      | case 1,
      |     Internal_Phase=0;
      |    Signal_PortWidth=1;
      |    Select1_Elements=[1 2];
      |    Select1_PortWidth=2;
      |    Select3_Elements=[1 2];
      |    Select3_PortWidth=4;
      | case 2,
      |     Internal_Phase=0;
      |     Signal_PortWidth=1;
      |     Select1_Elements=[1 2];
      |     Select1_PortWidth=2;
      |     Select3_Elements=[1 2 3 4];
      |     Select3_PortWidth=4;
      | case 3,
      |     Internal_Phase=[0 -2*pi/3 2*pi/3];
      |     Signal_PortWidth=3;
      |     Select1_Elements=[1 4 2 5 3 6];
      |     Select1_PortWidth=6;
      |    Select3_Elements=[1 2 3 4 5 6];
      |    Select3_PortWidth=12;
      | case 4,
      |     Internal_Phase=[0 -2*pi/3 2*pi/3];
      |     Signal_PortWidth=3;
      |     Select1_Elements=[1 4 2 5 3 6];
      |     Select1_PortWidth=6;
      |    Select3_Elements=[1 2 3 4 5 6 7 8 9 10 11 12];
      |    Select3_PortWidth=12;
      | end
      | power_initmask();
      mask Help:
      | The output pulses are a vector (with values=0 or 1). Depending on the selected "Generator Mode", the output vector contains:
      | For a 1-arm  bridge: Two pulses. Pulse 1 is for the upper switch and pulse 2 is for the lower switch.
      | For a 2-arm  bridge: Four pulses. Pulses 1 and 3 are respectively for the upper switches of the first and second arm. Pulses 2 and 4 are for the lower switches.
      | For a 3-arm  bridge: Six pulses. Pulses 1,3 and 5 are respectively for the upper switches of the first,second and third arm. Pulses 2,4 and 6 are for the lower switches.
      | For double 3-arm bridges: Twelve pulses.The first six pulses (pulses 1 to 6) must be sent to the first 3-arm bridge and the last six (pulses 7 to 12) to the second 3-arm bridge.
      | 
      | By selecting "Internal generation" you can can control the modulation index m, frequency and phase of the output voltage  from the internal parameters (m, Freq and Phase). Otherwise, external signals are used for pulse generation. The width of the input vector must be 1 for single phase bridges ( 1-arm or 2-arm)  and 3 for 3-phase bridges  (single or double bridge).
      mask TypeOptions GeneratorMode: 1-arm  bridge (2 pulses) | 2-arm  bridge (4 pulses) | 3-arm  bridge (6 pulses) | Double 3-arm  bridges (12 pulses)
      mask Callback Internal: powericon('psbcallbacks',gcb,'Discrete PWM Generator',[]);
  MI Controller : Subsystem
  Unit Delay4 : UnitDelay  SampleTime=Ts_Power  HasFrameUpgradeWarning=on
  VL-L_1 : Scope  NumInputPorts=2
  Vph_abc : Scope
  Vph_rms_1 : Scope
  u / m : Scope
  Pulses : Outport  VectorParamsAs1DForOutWhenUnconnected=off
  wires:
  MI Controller/2(u / m) -> u / m/1
  Unit Delay4/1 -> Pulses/1
  Discrete PWM Generator1/1(Pulses) -> Unit Delay4/1
  Bus Selector/1 -> Vph_abc/1, MI Controller/1(Vabc)  "<signal1>"
  Bus Selector/2 -> VL-L_1/1  "<signal2>"
  Bus Selector/3 -> VL-L_1/2  "<signal3>"
  Bus Selector/4 -> Vph_rms_1/1  "<signal4>"
  Means/1 -> Bus Selector/1
  MI Controller/1(Vabc_inv) -> Discrete PWM Generator1/1(Uref)

== system ACDCMG_woPV/Grid Bi-directional Converter 1.1 300 (DC) // 150 V (AC) P_nom 3kW1/Control of Inverter ==
  note: VL-L rms_1
  note: Primary control
  note: Control of Inverter
  Means : Inport
  Bus Selector : BusSelector  OutputSignals=signal1,signal2,signal3,signal4
  Discrete PWM Generator1 : Subsystem  AncestorBlock=|  DialogController=POWERSYS.PowerSysDialog  mask(Discrete PWM Generator){GeneratorMode=3-arm  bridge (6 pulses), Fc=4000, Ts=Ts_Power, Internal=off, mIndex=0.99, Freq=60, Phase=0}
      | powerlib_extras/Discrete 
      | Control Blocks/Discrete
      | PWM Generator
      mask prompts: GeneratorMode "Generator Mode"; Fc "Carrier frequency (Hz):"; Ts "Sample time:"; Internal "Internal generation of modulating signal(s)"; mIndex "Modulation index  (0<m<1) :"; Freq "Frequency of output voltage (Hz)"; Phase "Phase of output voltage (degrees)"
      mask help:
      | This discrete block generates pulses for carrier-based PWM (Pulse Width Modulation), self-commutated IGBTs,GTOs or FETs bridges.
      |
      | Depending on the number of bridge arms selected in the "Generator Mode" parameter, the block can be used either for single-phase or three-phase PWM control.
      mask init: same as ACDCMG_woPV/Grid Bi-directional Converter 1.1 300 (DC) // 150 V (AC) P_nom 3kW/Control of Inverter/Discrete PWM Generator1
      mask Help:
      | The output pulses are a vector (with values=0 or 1). Depending on the selected "Generator Mode", the output vector contains:
      | For a 1-arm  bridge: Two pulses. Pulse 1 is for the upper switch and pulse 2 is for the lower switch.
      | For a 2-arm  bridge: Four pulses. Pulses 1 and 3 are respectively for the upper switches of the first and second arm. Pulses 2 and 4 are for the lower switches.
      | For a 3-arm  bridge: Six pulses. Pulses 1,3 and 5 are respectively for the upper switches of the first,second and third arm. Pulses 2,4 and 6 are for the lower switches.
      | For double 3-arm bridges: Twelve pulses.The first six pulses (pulses 1 to 6) must be sent to the first 3-arm bridge and the last six (pulses 7 to 12) to the second 3-arm bridge.
      | 
      | By selecting "Internal generation" you can can control the modulation index m, frequency and phase of the output voltage  from the internal parameters (m, Freq and Phase). Otherwise, external signals are used for pulse generation. The width of the input vector must be 1 for single phase bridges ( 1-arm or 2-arm)  and 3 for 3-phase bridges  (single or double bridge).
      mask TypeOptions GeneratorMode: 1-arm  bridge (2 pulses) | 2-arm  bridge (4 pulses) | 3-arm  bridge (6 pulses) | Double 3-arm  bridges (12 pulses)
      mask Callback Internal: powericon('psbcallbacks',gcb,'Discrete PWM Generator',[]);
  MI Controller : Subsystem
  Unit Delay4 : UnitDelay  SampleTime=Ts_Power  HasFrameUpgradeWarning=on
  VL-L_1 : Scope  NumInputPorts=2
  Vph_abc : Scope
  Vph_rms_1 : Scope
  u / m : Scope
  Pulses : Outport  VectorParamsAs1DForOutWhenUnconnected=off
  wires:
  MI Controller/2(u / m) -> u / m/1
  Unit Delay4/1 -> Pulses/1
  Discrete PWM Generator1/1(Pulses) -> Unit Delay4/1
  Bus Selector/1 -> Vph_abc/1, MI Controller/1(Vabc)  "<signal1>"
  Bus Selector/2 -> VL-L_1/1  "<signal2>"
  Bus Selector/3 -> VL-L_1/2  "<signal3>"
  Bus Selector/4 -> Vph_rms_1/1  "<signal4>"
  Means/1 -> Bus Selector/1
  MI Controller/1(Vabc_inv) -> Discrete PWM Generator1/1(Uref)

== system ACDCMG_woPV/Grid Bi-directional Converter 1.1 300 (DC) // 150 V (AC) P_nom 3kW2/Control of Inverter ==
  note: VL-L rms_1
  note: Primary control
  note: Control of Inverter
  Means : Inport
  Bus Selector : BusSelector  OutputSignals=signal1,signal2,signal3,signal4
  Discrete PWM Generator1 : Subsystem  AncestorBlock=|  DialogController=POWERSYS.PowerSysDialog  mask(Discrete PWM Generator){GeneratorMode=3-arm  bridge (6 pulses), Fc=4000, Ts=Ts_Power, Internal=off, mIndex=0.99, Freq=60, Phase=0}
      | powerlib_extras/Discrete 
      | Control Blocks/Discrete
      | PWM Generator
      mask prompts: GeneratorMode "Generator Mode"; Fc "Carrier frequency (Hz):"; Ts "Sample time:"; Internal "Internal generation of modulating signal(s)"; mIndex "Modulation index  (0<m<1) :"; Freq "Frequency of output voltage (Hz)"; Phase "Phase of output voltage (degrees)"
      mask help:
      | This discrete block generates pulses for carrier-based PWM (Pulse Width Modulation), self-commutated IGBTs,GTOs or FETs bridges.
      |
      | Depending on the number of bridge arms selected in the "Generator Mode" parameter, the block can be used either for single-phase or three-phase PWM control.
      mask init: same as ACDCMG_woPV/Grid Bi-directional Converter 1.1 300 (DC) // 150 V (AC) P_nom 3kW/Control of Inverter/Discrete PWM Generator1
      mask Help:
      | The output pulses are a vector (with values=0 or 1). Depending on the selected "Generator Mode", the output vector contains:
      | For a 1-arm  bridge: Two pulses. Pulse 1 is for the upper switch and pulse 2 is for the lower switch.
      | For a 2-arm  bridge: Four pulses. Pulses 1 and 3 are respectively for the upper switches of the first and second arm. Pulses 2 and 4 are for the lower switches.
      | For a 3-arm  bridge: Six pulses. Pulses 1,3 and 5 are respectively for the upper switches of the first,second and third arm. Pulses 2,4 and 6 are for the lower switches.
      | For double 3-arm bridges: Twelve pulses.The first six pulses (pulses 1 to 6) must be sent to the first 3-arm bridge and the last six (pulses 7 to 12) to the second 3-arm bridge.
      | 
      | By selecting "Internal generation" you can can control the modulation index m, frequency and phase of the output voltage  from the internal parameters (m, Freq and Phase). Otherwise, external signals are used for pulse generation. The width of the input vector must be 1 for single phase bridges ( 1-arm or 2-arm)  and 3 for 3-phase bridges  (single or double bridge).
      mask TypeOptions GeneratorMode: 1-arm  bridge (2 pulses) | 2-arm  bridge (4 pulses) | 3-arm  bridge (6 pulses) | Double 3-arm  bridges (12 pulses)
      mask Callback Internal: powericon('psbcallbacks',gcb,'Discrete PWM Generator',[]);
  MI Controller : Subsystem
  Unit Delay4 : UnitDelay  SampleTime=Ts_Power  HasFrameUpgradeWarning=on
  VL-L_1 : Scope  NumInputPorts=2
  Vph_abc : Scope
  Vph_rms_1 : Scope
  u / m : Scope
  Pulses : Outport  VectorParamsAs1DForOutWhenUnconnected=off
  wires:
  MI Controller/2(u / m) -> u / m/1
  Unit Delay4/1 -> Pulses/1
  Discrete PWM Generator1/1(Pulses) -> Unit Delay4/1
  Bus Selector/1 -> Vph_abc/1, MI Controller/1(Vabc)  "<signal1>"
  Bus Selector/2 -> VL-L_1/1  "<signal2>"
  Bus Selector/3 -> VL-L_1/2  "<signal3>"
  Bus Selector/4 -> Vph_rms_1/1  "<signal4>"
  Means/1 -> Bus Selector/1
  MI Controller/1(Vabc_inv) -> Discrete PWM Generator1/1(Uref)
